simulink model "airbrakeSimulator"  (R2025b)
settings: Solver=FixedStepAuto  StartTime=0.0  StopTime=57  FixedStep=0.001  RelTol=1e-3
undefined symbols (not defined in the file): DiscIntNeverNeededParam
settings Model: Creator=esromabraham  LastModifiedBy=esromabraham

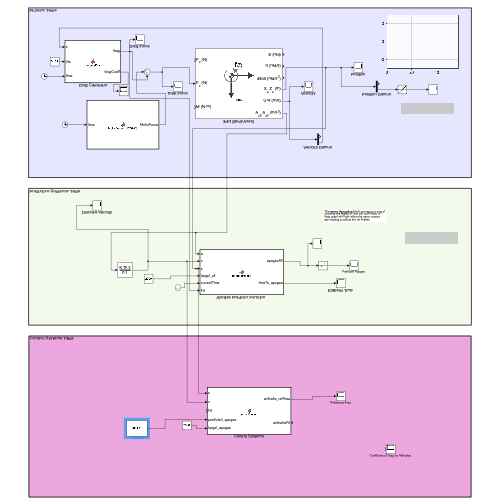
[thumbnail: Simulink's stored preview of the top-level diagram]
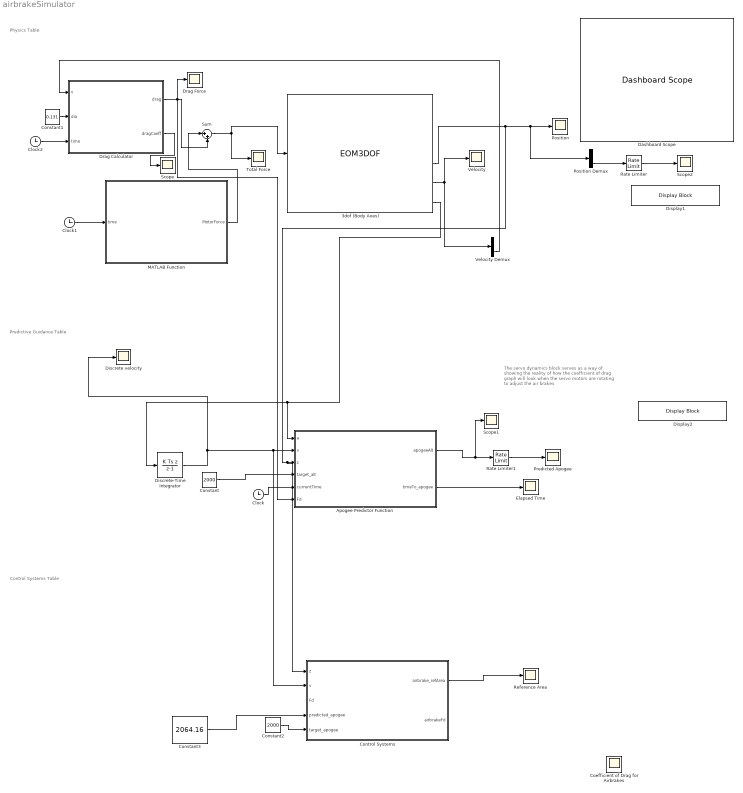
== system airbrakeSimulator ==
  note: Control Systems Table
  note: The servo dynamics block serves as a way of
      | showing the reality of how the coefficient of
      | drag graph will look when the servo motors
      | are rotating to adjust the air brakes
  note: Predictive Guidance Table
  note: Physics Table
  " Drag Calculator" : MATLAB Function  TreatAsAtomicUnit=on
  3dof (Body Axes) : EOM3DOF  v_ini=0  mass=13.576  g=-9.81
  "Apogee Predictor Function " : MATLAB Function  TreatAsAtomicUnit=on
  Clock : Clock
  Clock1 : Clock
  Clock2 : Clock
  Coefficient of Drag for Airbrakes : Scope
      settings: ActiveDisplayYMinimum=-1  ActiveDisplayYMaximum=1  DataLoggingVariableName=ScopeData7
  Constant : Constant  Value=2000
  Constant1 : Constant  Value=0.131
  Constant2 : Constant  Value=2000
  Constant3 : Constant  Value=2064.16
  Control Systems : MATLAB Function  TreatAsAtomicUnit=on
  Dashboard Scope : DashboardScope  FontColor=[0.0, 0.0, 0.0]
  Discrete velocity : Scope
      settings: ActiveDisplayYMinimum=291.97809991051849  ActiveDisplayYMaximum=312.46696240331539  DataLoggingVariableName=ScopeData8
  Discrete-Time Integrator : DiscreteIntegrator  IntegratorMethod=Integration: Backward Euler  SampleTime=-1  ICPrevOutput=DiscIntNeverNeededParam  ICPrevScaledInput=DiscIntNeverNeededParam
  Display1 : DisplayBlock  LabelPosition=Hide  Format=bank  Transparency=1  GridColor=[0.502, 0.502, 0.502]
  Display2 : DisplayBlock  LabelPosition=Hide  Format=bank  Transparency=1  GridColor=[0.502, 0.502, 0.502]
  Drag Force : Scope
      settings: ActiveDisplayYMinimum=-1  ActiveDisplayYMaximum=1  DataLoggingVariableName=ScopeData3
  Elapsed Time : Scope
      settings: ActiveDisplayYMinimum=4.5521033385037128  ActiveDisplayYMaximum=13.087344302359135  DataLoggingVariableName=ScopeData6
  MATLAB Function : MATLAB Function  TreatAsAtomicUnit=on
  Position : Scope
      settings: ActiveDisplayYMinimum=-251.20533671943687  ActiveDisplayYMaximum=2260.8480304749323
  Position Demux : Demux  Outputs=2
  "Predicted Apogee " : Scope
      settings: ActiveDisplayYMinimum=-254.84305290405223  ActiveDisplayYMaximum=2292.7929489685152  DataLoggingVariableName=ScopeData9
  Rate Limiter : RateLimiter  RisingSlewLimit=9999999999  FallingSlewLimit=0  SampleTimeMode=inherited
  Rate Limiter1 : RateLimiter  RisingSlewLimit=999999999  FallingSlewLimit=0  SampleTimeMode=inherited
  Reference Area : Scope
      settings: ActiveDisplayYMinimum=-0.095738392045454535  ActiveDisplayYMaximum=0.5298853579545455  DataLoggingVariableName=ScopeData11
  Scope : Scope
      settings: ActiveDisplayYMinimum=-1  ActiveDisplayYMaximum=1  DataLoggingVariableName=ScopeData5
  Scope1 : Scope
      settings: ActiveDisplayYMinimum=-3088.7086594080656  ActiveDisplayYMaximum=2636.6963947761769  DataLoggingVariableName=ScopeData4
  Scope2 : Scope
      settings: DataLoggingVariableName=ScopeData10
  Sum : Sum  Inputs=|++
  Total Force : Scope
      settings: ActiveDisplayYMinimum=-1  ActiveDisplayYMaximum=1  DataLoggingVariableName=ScopeData2
  Velocity : Scope
      settings: ActiveDisplayYMinimum=-1  ActiveDisplayYMaximum=1
  Velocity Demux : Demux  Outputs=2
  wires:
  3dof (Body Axes)/5 -> Velocity/1, Velocity Demux/1
  3dof (Body Axes)/4 -> "Apogee Predictor Function "/3(z), Control Systems/1(z), Position Demux/1, Position/1
  MATLAB Function/1(MotorForce) -> Sum/1
  " Drag Calculator"/1(drag) -> Sum/2, Drag Force/1, "Apogee Predictor Function "/6(Fd)
  Sum/1 -> 3dof (Body Axes)/2, Total Force/1
  Velocity Demux/2 -> " Drag Calculator"/1(v)
  Position Demux/2 -> Rate Limiter/1
  Rate Limiter/1 -> Scope2/1
  "Apogee Predictor Function "/2(timeTo_apogee) -> Elapsed Time/1
  Constant/1 -> "Apogee Predictor Function "/4(target_alt)
  Clock/1 -> "Apogee Predictor Function "/5(currentTime)
  3dof (Body Axes)/6 -> "Apogee Predictor Function "/1(a), Discrete-Time Integrator/1
  "Apogee Predictor Function "/1(apogeeAlt) -> Scope1/1, Rate Limiter1/1
  Rate Limiter1/1 -> "Predicted Apogee "/1
  Clock1/1 -> MATLAB Function/1(time)
  Clock2/1 -> " Drag Calculator"/3(time)
  " Drag Calculator"/2(dragCoeff) -> Scope/1
  Constant1/1 -> " Drag Calculator"/2(dia)
  Control Systems/1(airbrake_refArea) -> Reference Area/1
  Constant2/1 -> Control Systems/5(target_apogee)
  Constant3/1 -> Control Systems/4(predicted_apogee)
  Discrete-Time Integrator/1 -> "Apogee Predictor Function "/2(v), Control Systems/2(v), Discrete velocity/1

== matlab function airbrakeSimulator/Apogee Predictor Function  ==
  data: a input; v input; z input; target_alt input; currentTime input; apogeeAlt output; timeTo_apogee output; Fd input
function [apogeeAlt, timeTo_apogee] = apogeePredict(a, v, z, target_alt, currentTime, Fd)

% V is the velocity vector, with 2 components, U  being the x-velocity, and w being the z-velocity
% a is acceleration
% v is velocity
% z is the position in the z-axis


currentAlt = z(2);
currentVelocity = v(2);
currentAcceleration = a(2);


m = 13.576; % in kg
v_sim = currentVelocity;
alt_sim = currentAlt;
a_sim = currentAcceleration;
t = currentTime;
deltaT = 0.001; % changing it by x10 doesn't   
apogeeAlt = 0; % we are leaving this as an empty value
timeTo_apogee = 20.6; % time it takes to get to apogee




for i = 1:1000
    F = -Fd(i/i) - (9.81*m);
    
    a_sim = F/m;
    v_sim = v_sim + a_sim*deltaT;
    alt_sim = alt_sim + v_sim*deltaT;
    t = t + deltaT;

    apogeeAlt = alt_sim;


    if apogeeAlt-target_alt <= 2
        break;
    end
end

== matlab function airbrakeSimulator/ Drag Calculator ==
  data: drag output; v input; dia input; time input; dragCoeff output
function [drag, dragCoeff]= computeDrag(v, dia, time)

A = pi * (dia/2)^2;
rho = 1.2;

y_data=[1.206
0.555
0.494
0.464
0.445
0.431
0.421
0.412
0.411
0.411
0.411
0.411
0.411
0.411
0.411
0.411
0.411
0.412
0.412
0.412
0.412
0.412
0.412
0.412
0.412
0.413
0.413
0.413
0.413
0.413
0.413
0.414
0.414
0.414
0.414
0.415
0.415
0.415
0.415
0.415
0.416
0.416
0.416
0.416
0.417
0.417
0.417
0.418
0.418
0.418
0.419
0.419
0.419
0.42
0.42
0.42
0.421
0.421
0.421
0.422
0.422
0.422
0.423
0.423
0.424
0.424
0.425
0.425
0.425
0.426
0.426
0.427
0.427
0.428
0.428
0.429
0.429
0.43
0.43
0.431
0.431
0.432
0.432
0.433
0.433
0.434
0.435
0.435
0.436
0.436
0.437
0.437
0.438
0.439
0.439
0.44
0.441
0.441
0.442
0.443
0.443
0.444
0.445
0.445
0.446
0.447
0.448
0.448
0.449
0.45
0.451
0.451
0.452
0.453
0.454
0.455
0.455
0.456
0.457
0.458
0.459
0.46
0.46
0.461
0.462
0.463
0.464
0.465
0.466
0.467
0.468
0.469
0.47
0.471
0.472
0.473
0.474
0.475
0.476
0.477
0.478
0.479
0.481
0.482
0.483
0.484
0.485
0.487
0.488
0.489
0.49
0.492
0.493
0.494
0.496
0.497
0.498
0.5
0.501
0.503
0.504
0.506
0.508
0.509
0.511
0.513
0.514
0.516
0.518
0.52
0.522
0.524
0.526
0.528
0.53
0.533
0.535
0.537
0.54
0.543
0.546
0.546
0.546
0.546
0.546
0.546
0.546
0.546
0.546
0.546
0.547
0.547
0.547
0.547
0.547
0.547
0.547
0.548
0.548
0.548
0.548
0.554
0.559
0.564
0.57
0.573
0.577
0.58
0.584
0.586
0.587
0.589
0.591
0.591
0.591
0.591
0.592
0.591
0.589
0.588
0.587
0.586
0.584
0.582
0.58
0.577
0.575
0.572
0.569
0.566
0.563
0.559
0.556
0.552
0.548
0.545
0.541
0.537
0.533
0.529
0.525

];
x_data=[0
1.715
3.43
5.145
6.86
8.575
10.29
12.005
13.72
15.435
17.15
18.865
20.58
22.295
24.01
25.725
27.44
29.155
30.87
32.585
34.3
36.015
37.73
39.445
41.16
42.875
44.59
46.305
48.02
49.735
51.45
53.165
54.88
56.595
58.31
60.025
61.74
63.455
65.17
66.885
68.6
70.315
72.03
73.745
75.46
77.175
78.89
80.605
82.32
84.035
85.75
87.465
89.18
90.895
92.61
94.325
96.04
97.755
99.47
101.185
102.9
104.615
106.33
108.045
109.76
111.475
113.19
114.905
116.62
118.335
120.05
121.765
123.48
125.195
126.91
128.625
130.34
132.055
133.77
135.485
137.2
138.915
140.63
142.345
144.06
145.775
147.49
149.205
150.92
152.635
154.35
156.065
157.78
159.495
161.21
162.925
164.64
166.355
168.07
169.785
171.5
173.215
174.93
176.645
178.36
180.075
181.79
183.505
185.22
186.935
188.65
190.365
192.08
193.795
195.51
197.225
198.94
200.655
202.37
204.085
205.8
207.515
209.23
210.945
212.66
214.375
216.09
217.805
219.52
221.235
222.95
224.665
226.38
228.095
229.81
231.525
233.24
234.955
236.67
238.385
240.1
241.815
243.53
245.245
246.96
248.675
250.39
252.105
253.82
255.535
257.25
258.965
260.68
262.395
264.11
265.825
267.54
269.255
270.97
272.685
274.4
276.115
277.83
279.545
281.26
282.975
284.69
286.405
288.12
289.835
291.55
293.265
294.98
296.695
298.41
300.125
301.84
303.555
305.27
306.985
308.7
310.415
312.13
313.845
315.56
317.275
318.99
320.705
322.42
324.135
325.85
327.565
329.28
330.995
332.71
334.425
336.14
337.855
339.57
341.285
343
344.715
346.43
348.145
349.86
351.575
353.29
355.005
356.72
358.435
360.15
361.865
363.58
365.295
367.01
368.725
370.44
372.155
373.87
375.585
377.3
379.015
380.73
382.445
384.16
385.875
387.59
389.305
391.02
392.735
394.45
396.165
397.88
399.595
401.31
403.025
404.74
406.455
408.17
409.885
411.6
];

if (abs(v) <x_data(end))
    dragCoeff = interp1(x_data, y_data, abs(v), 'linear');
    drag = A * dragCoeff * 0.5 * rho * -v*abs(v);

else
    dragCoeff = 0;
    drag = 0;


end
%#codegen

== matlab function airbrakeSimulator/MATLAB Function ==
  data: time input; MotorForce output
function MotorForce = MotorForce_L1256WS(time)
y_data=[0
13.86513022
1220.003521
1400.239753
1439.078899
1469.660692
1466.083402
1445.399674
1340.958951
1231.08505
1098.456359
1064.1
829.7292739
376.0321
55.77052487
28.0667017
0
];
x_data=[0
0.017
0.045
0.19
0.465
0.77
1.076
1.381
1.723
2.029
2.485
2.71
2.788
2.939
3.023
3.041
3.059
];
if (time <x_data(end))
    MotorForce = interp1(x_data, y_data, time, 'linear');

else
    MotorForce = 0;
end
%#codegen

== matlab function airbrakeSimulator/Control Systems ==
  data: z input; v input; Fd input; predicted_apogee input; target_apogee input; airbrake_refArea output; airbrakeFd output
function [airbrake_refArea, airbrakeFd] = controlSystem(z, v, Fd, predicted_apogee, target_apogee)

m = 13.576;
rho = 1.225;
g = -9.81;
airbrake_maxArea = 0.05;
airbrake_Cd = 0.4; % I will make a guess here, but I will change this later

position = z(2);
acceleration = a(2);
velocity = v(2);





overshoot = predicted_apogee - target_apogee;

remaining_distance = target_apogee - position;

if predicted_apogee > target_apogee && overshoot ~= 0
